simulink model "Test_model_Function_3_12_64"  (R2024a)
settings: Solver=VariableStepAuto  StartTime=0.0  StopTime=inf  RelTol=1e-3
undefined symbols (not defined in the file or in its folder): X, Y, Z
libraries: sm_lib x62, nesl_utility x21, robotcorelib x4
(part 1 of 3)
settings Model: Creator=pimna  LastModifiedBy=Chaiyapat Gotji

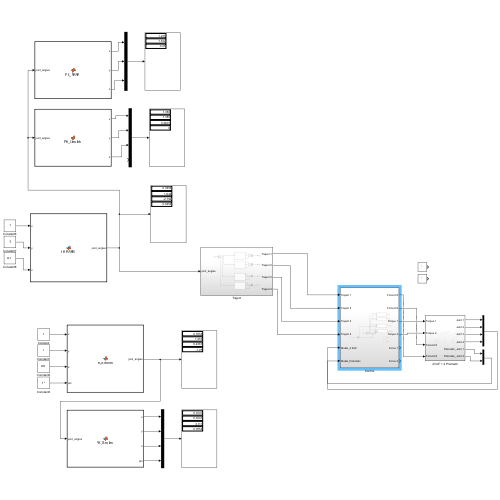
[thumbnail: Simulink's stored preview of the top-level diagram]
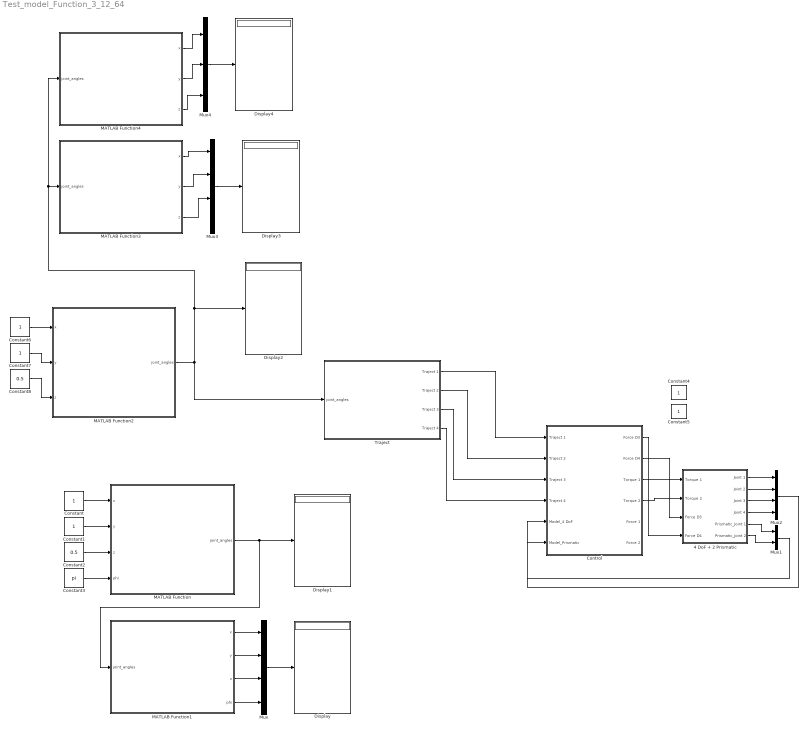
== system Test_model_Function_3_12_64 ==
  4 DoF + 2 Prismatic : Subsystem
  Constant{,1,6..7} (4 alike) : Constant  VectorParams1D=off  SampleTime=-1
  Constant2 : Constant  Value=0.5  VectorParams1D=off  SampleTime=-1
  Constant3 : Constant  Value=pi  VectorParams1D=off  SampleTime=-1
  Constant4 : Constant
  Constant5 : Constant
  Constant8 : Constant  Value=0.5  VectorParams1D=off  SampleTime=-1
  Control : Subsystem
  Display{,1..4} (5 alike) : Display
  MATLAB Function : MATLAB Function  TreatAsAtomicUnit=on
  MATLAB Function1 : MATLAB Function  TreatAsAtomicUnit=on
  MATLAB Function2 : MATLAB Function  TreatAsAtomicUnit=on
  MATLAB Function3 : MATLAB Function  TreatAsAtomicUnit=on
  MATLAB Function4 : MATLAB Function  TreatAsAtomicUnit=on
  Mux : Mux
  Mux1 : Mux  Inputs=2
  Mux2 : Mux
  Mux3 : Mux
  Mux4 : Mux  Inputs=3
  Traject : Subsystem
  wires:
  MATLAB Function1/2(y) -> Mux/2
  MATLAB Function1/4(phi) -> Mux/4
  MATLAB Function1/1(x) -> Mux/1
  MATLAB Function/1(joint_angles) -> MATLAB Function1/1(joint_angles), Display1/1
  Mux/1 -> Display/1
  MATLAB Function1/3(z) -> Mux/3
  Constant2/1 -> MATLAB Function/3(z)
  Constant3/1 -> MATLAB Function/4(phi)
  4 DoF + 2 Prismatic/6(Prismatic_Joint 2) -> Mux1/2
  Constant/1 -> MATLAB Function/1(x)
  4 DoF + 2 Prismatic/4(Joint 4) -> Mux2/4
  4 DoF + 2 Prismatic/5(Prismatic_Joint 1) -> Mux1/1
  Mux1/1 -> Control/6(Model_Prismatic)
  4 DoF + 2 Prismatic/1(Joint 1) -> Mux2/1
  Constant1/1 -> MATLAB Function/2(y)
  4 DoF + 2 Prismatic/2(Joint 2) -> Mux2/2
  Mux2/1 -> Control/5(Model_4 DoF)
  4 DoF + 2 Prismatic/3(Joint 3) -> Mux2/3
  Control/3(Torque 1) -> 4 DoF + 2 Prismatic/1(Torque 1)
  Control/4(Torque 2) -> 4 DoF + 2 Prismatic/2(Torque 2)
  Traject/1(Traject 1) -> Control/1(Traject 1)
  Traject/2(Traject 2) -> Control/2(Traject 2)
  Traject/3(Traject 3) -> Control/3(Traject 3)
  Traject/4(Traject 4) -> Control/4(Traject 4)
  Control/2(Force D4) -> 4 DoF + 2 Prismatic/3(Force D3)
  Control/1(Force D3) -> 4 DoF + 2 Prismatic/4(Force D4)
  Constant6/1 -> MATLAB Function2/1(x)
  Constant7/1 -> MATLAB Function2/2(y)
  Constant8/1 -> MATLAB Function2/3(z)
  MATLAB Function2/1(joint_angles) -> Traject/1(joint_angles), MATLAB Function4/1(joint_angles), MATLAB Function3/1(joint_angles), Display2/1
  MATLAB Function3/3(z) -> Mux3/3
  Mux3/1 -> Display3/1
  MATLAB Function3/2(y) -> Mux3/2
  MATLAB Function3/1(x) -> Mux3/1
  Mux4/1 -> Display4/1
  MATLAB Function4/1(x) -> Mux4/1
  MATLAB Function4/2(y) -> Mux4/2
  MATLAB Function4/3(z) -> Mux4/3
